simulink model "PDQuadrotor_with_the_position_control"  (R2015b)
settings: Solver=VariableStepAuto  StartTime=start_simulation_drone  StopTime=end_simulation_drone  RelTol=1e-3
values from neighbouring files (symbols this model uses):
  b = 3.13*10^(-5)    (= 3.13e-05)    [drone_parameters.m]    (also in simulazione_sistema.m)
  C_10 = 0.5    [controller_parameters.m]    (also in controller_paramters.m; simulazione_sistema.m)
  C_11 = 2    [controller_parameters.m]    (also in controller_paramters.m; simulazione_sistema.m)
  C_12 = 0.5    [controller_parameters.m]    (also in controller_paramters.m; simulazione_sistema.m)
  C_9 = 2    [controller_parameters.m]    (also in controller_paramters.m; simulazione_sistema.m)
  chi_5_pre = 0    [controller_parameters.m]    (also in controller_paramters.m; drone_model.m = chi_5(end))
  chi_6_pre = 0    [controller_parameters.m]    (also in controller_paramters.m; drone_model.m = chi_6(end))
  d = 7.5*10^(-7)    (= 7.5e-07)    [drone_parameters.m]    (also in simulazione_sistema.m)
  g = 9.81    [drone_parameters.m]    (also in simulazione_sistema.m)
  Ix = 7.5*10^(-3)    (= 0.0075)    [drone_parameters.m]    (also in simulazione_sistema.m)
  Iy = 7.5*10^(-3)    (= 0.0075)    [drone_parameters.m]    (also in simulazione_sistema.m)
  Iz = 1.3*10^(-2)    (= 0.013)    [drone_parameters.m]    (also in simulazione_sistema.m)
  Jr = 6.5*10^(-5)    (= 6.5e-05)    [drone_parameters.m]    (also in simulazione_sistema.m)
  kdp = 0.4e1    (= 4)    [controller_parameters.m]    (also in controller_paramters.m; simulazione_sistema.m)
  kdps = 0.4e1    (= 4)    [controller_parameters.m]    (also in controller_paramters.m; simulazione_sistema.m)
  kdt = 0.4e1    (= 4)    [controller_parameters.m]    (also in controller_paramters.m; simulazione_sistema.m)
  kdz = 20e1    (= 200)    [controller_parameters.m]    (also in controller_paramters.m; simulazione_sistema.m)
  kpp = 0.8e1    (= 8)    [controller_parameters.m]    (also in controller_paramters.m; simulazione_sistema.m)
  kpps = 1e1    (= 10)    [controller_parameters.m]    (also in controller_paramters.m; simulazione_sistema.m)
  kpt = 1.2e1    (= 12)    [controller_parameters.m]    (also in controller_paramters.m; simulazione_sistema.m)
  kpz = 100e1    (= 1000)    [controller_parameters.m]    (also in controller_paramters.m; simulazione_sistema.m)
  l = 0.23    [drone_parameters.m]    (also in simulazione_sistema.m)
  lambda_5 = 0.025    [controller_parameters.m]    (also in controller_paramters.m; simulazione_sistema.m)
  lambda_6 = 0.025    [controller_parameters.m]    (also in controller_paramters.m; simulazione_sistema.m)
  m = 0.65    [drone_parameters.m]    (also in simulazione_sistema.m)
  phi_dot_pre = 0    [controller_parameters.m]    (also in controller_paramters.m; drone_model.m = phi_dot(end))
  pitch_regulator_pre = pitch_initial    [controller_parameters.m]    (also in controller_paramters.m)
  psi_dot_pre = 0    [controller_parameters.m]    (also in controller_paramters.m; drone_model.m = psi_dot(end))
  roll_regulator_pre = roll_initial    [controller_parameters.m]    (also in controller_paramters.m)
  theta_dot_pre = 0    [controller_parameters.m]    (also in controller_paramters.m; drone_model.m = theta_dot(end))
  x_dot_pre = 0    [controller_parameters.m]    (also in drone_model.m = x_dot(end))
  x_next_drone = x_next    [drone_model.m]
  x_next_pre = x_next    [controller_parameters.m]    (also in drone_model.m = x_meas(end))
  y_dot_pre = 0    [controller_parameters.m]    (also in drone_model.m = y_dot(end))
  y_next_drone = -z_next    [drone_model.m]
  y_next_pre = -z_next    [controller_parameters.m]    (also in drone_model.m = y_meas(end))
  yaw_regulator = delta_yaw_regulator + yaw_initial    [drone_control.m]
  yaw_regulator_pre = yaw_initial    [controller_parameters.m]    (also in controller_paramters.m)
  z_dot_pre = 0    [controller_parameters.m]    (also in drone_model.m = z_dot(end))
  z_next_drone = y_next    [drone_model.m]
  z_next_pre = y_next    [controller_parameters.m]    (also in drone_model.m = z_meas(end))
settings Model: Creator=Giuseppe  LastModifiedBy=giuse

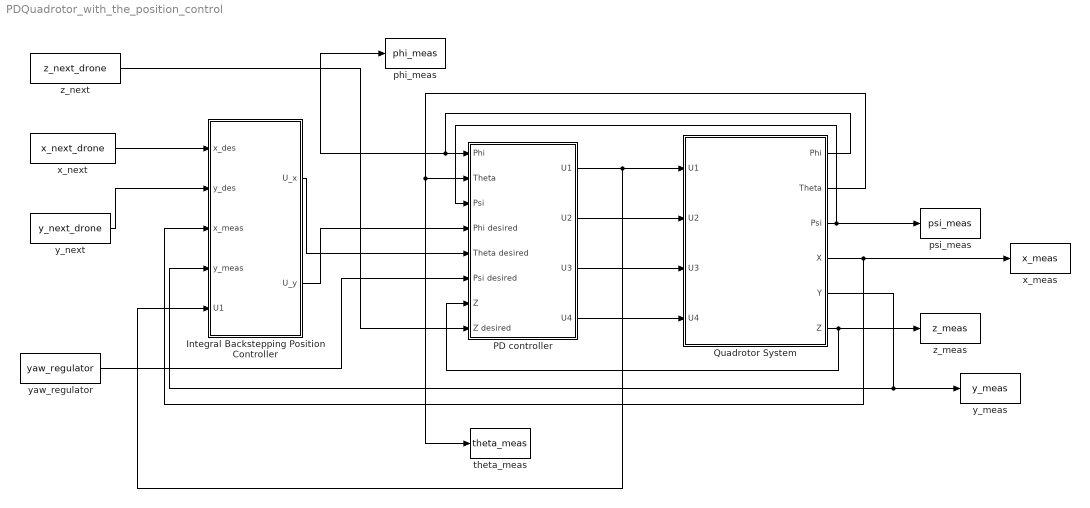
== system PDQuadrotor_with_the_position_control ==
  Integral Backstepping Position Controller : Subsystem
  PD controller : Subsystem
  Quadrotor System : Subsystem
  phi_meas : ToWorkspace  VariableName=phi_meas  SampleTime=-1
  psi_meas : ToWorkspace  VariableName=psi_meas  SampleTime=-1
  theta_meas : ToWorkspace  VariableName=theta_meas  SampleTime=-1
  "x_meas " : ToWorkspace  VariableName=x_meas  SampleTime=-1
  x_next : Constant  Value=x_next_drone
  y_meas : ToWorkspace  VariableName=y_meas  SampleTime=-1
  y_next : Constant  Value=y_next_drone
  yaw_regulator : Constant  Value=yaw_regulator
  z_meas : ToWorkspace  VariableName=z_meas  SampleTime=-1
  z_next : Constant  Value=z_next_drone
  wires:
  PD controller/1(U1) -> Integral Backstepping Position Controller/5(U1), Quadrotor System/1(U1)
  PD controller/2(U2) -> Quadrotor System/2(U2)
  PD controller/3(U3) -> Quadrotor System/3(U3)
  PD controller/4(U4) -> Quadrotor System/4(U4)
  Quadrotor System/6(Z) -> PD controller/7(Z), z_meas/1
  Quadrotor System/1(Phi) -> PD controller/1(Phi), phi_meas/1
  Quadrotor System/2(Theta) -> theta_meas/1, PD controller/2(Theta)
  Quadrotor System/3(Psi) -> PD controller/3(Psi), psi_meas/1
  Integral Backstepping Position Controller/2(U_y) -> PD controller/4(Phi desired)
  Integral Backstepping Position Controller/1(U_x) -> PD controller/5(Theta desired)
  z_next/1 -> PD controller/8(Z desired)
  Quadrotor System/5(Y) -> Integral Backstepping Position Controller/4(y_meas), y_meas/1
  yaw_regulator/1 -> PD controller/6(Psi desired)
  y_next/1 -> Integral Backstepping Position Controller/2(y_des)
  x_next/1 -> Integral Backstepping Position Controller/1(x_des)
  Quadrotor System/4(X) -> Integral Backstepping Position Controller/3(x_meas), "x_meas "/1

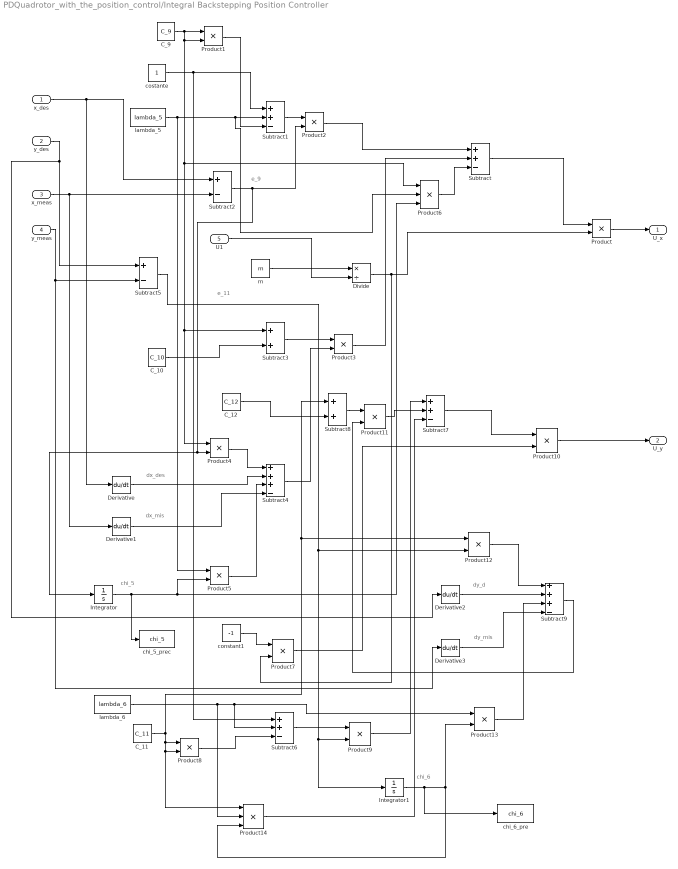
== system PDQuadrotor_with_the_position_control/Integral Backstepping Position Controller ==
  note: chi_6
  note: dy_mis
  note: dy_d
  note: e_11
  note: chi_5
  note: dx_des
  note: dx_mis
  note: e_9
  x_des : Inport
  y_des : Inport  Port=2
  x_meas : Inport  Port=3
  y_meas : Inport  Port=4
  U1 : Inport  Port=5
  C_10 : Constant  Value=C_10
  C_11 : Constant  Value=C_11
  C_12 : Constant  Value=C_12
  C_9 : Constant  Value=C_9
  Derivative{,1..3} (4 alike) : Derivative
  Divide : Product  Inputs=*/
  Integrator : Integrator  InitialCondition=chi_5_pre
  Integrator1 : Integrator  InitialCondition=chi_6_pre
  Product{,1..5,7..13} (13 alike) : Product
  Product14 : Product  Inputs=3
  Product6 : Product  Inputs=3
  Subtract{,1,6..7} (4 alike) : Sum  Inputs=++-
  Subtract2 : Sum  Inputs=+-
  Subtract3 : Sum
  Subtract4 : Sum  Inputs=+++-
  Subtract5 : Sum  Inputs=+-
  Subtract8 : Sum
  Subtract9 : Sum  Inputs=+++-
  chi_5_prec : ToWorkspace  VariableName=chi_5  SampleTime=-1
  chi_6_pre : ToWorkspace  VariableName=chi_6  SampleTime=-1
  constant1 : Constant  Value=-1
  costante : Constant
  lambda_5 : Constant  Value=lambda_5
  lambda_6 : Constant  Value=lambda_6
  m : Constant  Value=m
  U_x : Outport
  U_y : Outport  Port=2
  wires:
  m/1 -> Divide/1
  U1/1 -> Divide/2
  Divide/1 -> Product7/2, Product/2
  Subtract/1 -> Product/1
  costante/1 -> Subtract6/1, Subtract1/1
  lambda_5/1 -> Product6/2, Subtract1/2, Product5/1
  C_9/1 -> Product6/1, Subtract3/1, Product4/1, Product1/2, Product1/1
  Product1/1 -> Subtract1/3
  Subtract1/1 -> Product2/1
  Subtract2/1 -> Integrator/1, Product4/2, Product2/2
  x_des/1 -> Derivative/1, Subtract2/1
  x_meas/1 -> Derivative1/1, Subtract2/2
  Product2/1 -> Subtract/1
  Subtract3/1 -> Product3/1
  C_10/1 -> Subtract3/2
  Subtract4/1 -> Product3/2
  Product4/1 -> Subtract4/1
  Derivative/1 -> Subtract4/2
  Derivative1/1 -> Subtract4/4
  Product5/1 -> Subtract4/3
  Integrator/1 -> chi_5_prec/1, Product6/3, Product5/2
  Product3/1 -> Subtract/2
  Product/1 -> U_x/1
  Product6/1 -> Subtract/3
  constant1/1 -> Product7/1
  C_11/1 -> Product12/1, Subtract8/1, Product14/1, Product8/2, Product8/1
  Product8/1 -> Subtract6/3
  lambda_6/1 -> Product14/2, Subtract6/2, Product13/1
  Subtract6/1 -> Product9/1
  y_des/1 -> Subtract5/1, Derivative2/1
  y_meas/1 -> Subtract5/2, Derivative3/1
  Subtract5/1 -> Product12/2, Product9/2, Integrator1/1
  Product10/1 -> U_y/1
  Subtract7/1 -> Product10/1
  Product7/1 -> Product10/2
  Product9/1 -> Subtract7/1
  C_12/1 -> Subtract8/2
  Subtract8/1 -> Product11/1
  Product11/1 -> Subtract7/2
  Subtract9/1 -> Product11/2
  Product12/1 -> Subtract9/1
  Derivative2/1 -> Subtract9/2
  Derivative3/1 -> Subtract9/4
  Product13/1 -> Subtract9/3
  Integrator1/1 -> chi_6_pre/1, Product14/3, Product13/2
  Product14/1 -> Subtract7/3

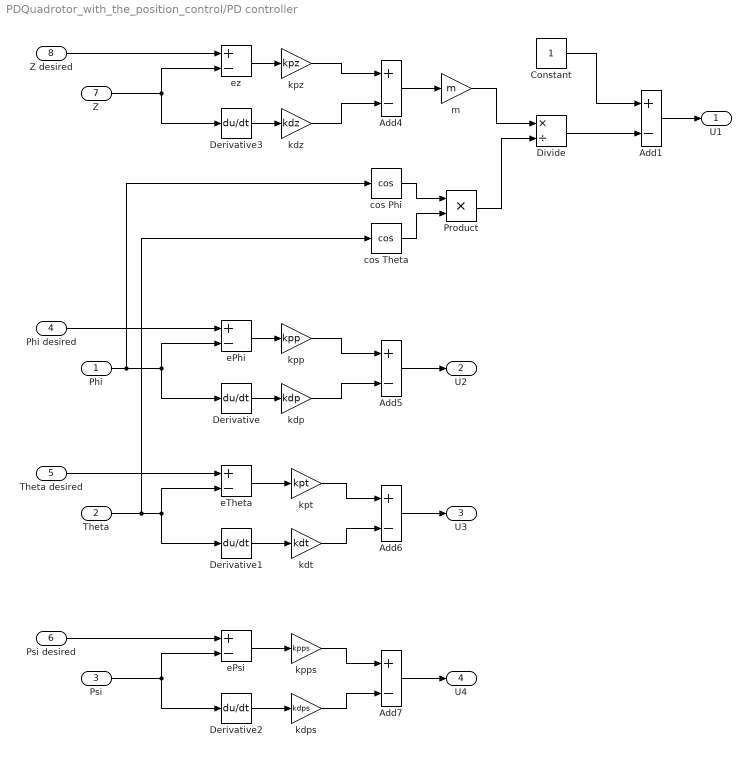
== system PDQuadrotor_with_the_position_control/PD controller ==
  Phi : Inport
  Theta : Inport  Port=2
  Psi : Inport  Port=3
  Phi desired : Inport  Port=4
  Theta desired : Inport  Port=5
  Psi desired : Inport  Port=6
  Z : Inport  Port=7
  Z desired : Inport  Port=8
  Add{1,4..7} (5 alike) : Sum  Inputs=+-
  Constant : Constant
  Derivative{,1..3} (4 alike) : Derivative
  Divide : Product  Inputs=*/
  Product : Product  RndMeth=Zero
  cos Phi : Trigonometry  Operator=cos
  cos Theta : Trigonometry  Operator=cos
  ePhi : Sum  Inputs=+-
  ePsi : Sum  Inputs=+-
  eTheta : Sum  Inputs=+-
  ez : Sum  Inputs=+-
  kdp : Gain  Gain=kdp
  kdps : Gain  Gain=kdps
  kdt : Gain  Gain=kdt
  kdz : Gain  Gain=kdz
  kpp : Gain  Gain=kpp
  kpps : Gain  Gain=kpps
  kpt : Gain  Gain=kpt
  kpz : Gain  Gain=kpz
  m : Gain  Gain=m
  U1 : Outport
  U2 : Outport  Port=2
  U3 : Outport  Port=3
  U4 : Outport  Port=4
  wires:
  Phi/1 -> Derivative/1, ePhi/2, cos Phi/1
  Theta/1 -> Derivative1/1, eTheta/2, cos Theta/1
  Psi/1 -> Derivative2/1, ePsi/2
  Phi desired/1 -> ePhi/1
  Theta desired/1 -> eTheta/1
  Psi desired/1 -> ePsi/1
  ePhi/1 -> kpp/1
  Derivative/1 -> kdp/1
  eTheta/1 -> kpt/1
  Derivative1/1 -> kdt/1
  ePsi/1 -> kpps/1
  Derivative2/1 -> kdps/1
  Z/1 -> Derivative3/1, ez/2
  Z desired/1 -> ez/1
  ez/1 -> kpz/1
  Derivative3/1 -> kdz/1
  kpz/1 -> Add4/1
  kdz/1 -> Add4/2
  kpp/1 -> Add5/1
  kdp/1 -> Add5/2
  Add5/1 -> U2/1
  kpt/1 -> Add6/1
  kdt/1 -> Add6/2
  Add6/1 -> U3/1
  kpps/1 -> Add7/1
  kdps/1 -> Add7/2
  Add7/1 -> U4/1
  cos Phi/1 -> Product/1
  cos Theta/1 -> Product/2
  Add4/1 -> m/1
  m/1 -> Divide/1
  Product/1 -> Divide/2
  Constant/1 -> Add1/1
  Divide/1 -> Add1/2
  Add1/1 -> U1/1

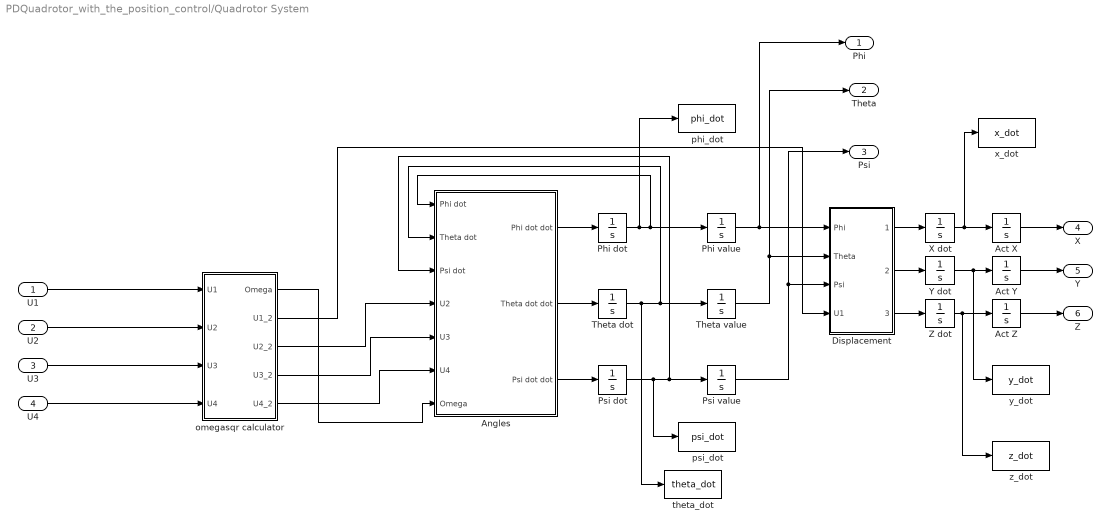
== system PDQuadrotor_with_the_position_control/Quadrotor System ==
  U1 : Inport
  U2 : Inport  Port=2
  U3 : Inport  Port=3
  U4 : Inport  Port=4
  Act X : Integrator  InitialCondition=x_next_pre
  Act Y : Integrator  InitialCondition=y_next_pre
  Act Z : Integrator  InitialCondition=z_next_pre
  Angles : Subsystem
  Displacement : Subsystem
  Phi dot : Integrator  InitialCondition=phi_dot_pre
  Phi value : Integrator  InitialCondition=roll_regulator_pre  ZeroCross=off
  Psi dot : Integrator  InitialCondition=psi_dot_pre  ZeroCross=off
  Psi value : Integrator  InitialCondition=yaw_regulator_pre  ZeroCross=off
  Theta dot : Integrator  InitialCondition=theta_dot_pre  ZeroCross=off
  Theta value : Integrator  InitialCondition=pitch_regulator_pre  ZeroCross=off
  X dot : Integrator  InitialCondition=x_dot_pre
  Y dot : Integrator  InitialCondition=y_dot_pre
  Z dot : Integrator  InitialCondition=z_dot_pre
  omegasqr calculator : Subsystem
  phi_dot : ToWorkspace  VariableName=phi_dot  SampleTime=-1
  psi_dot : ToWorkspace  VariableName=psi_dot  SampleTime=-1
  theta_dot : ToWorkspace  VariableName=theta_dot  SampleTime=-1
  x_dot : ToWorkspace  VariableName=x_dot  SampleTime=-1
  y_dot : ToWorkspace  VariableName=y_dot  SampleTime=-1
  z_dot : ToWorkspace  VariableName=z_dot  SampleTime=-1
  Phi : Outport
  Theta : Outport  Port=2
  Psi : Outport  Port=3
  X : Outport  Port=4
  Y : Outport  Port=5
  Z : Outport  Port=6
  wires:
  Angles/1(Phi dot dot) -> Phi dot/1
  Angles/2(Theta dot dot) -> Theta dot/1
  Angles/3(Psi dot dot) -> Psi dot/1
  Phi dot/1 -> Phi value/1, Angles/1(Phi dot), phi_dot/1
  Theta dot/1 -> Theta value/1, Angles/2(Theta dot), theta_dot/1
  Psi dot/1 -> Psi value/1, Angles/3(Psi dot), psi_dot/1
  omegasqr calculator/3(U2_2) -> Angles/4(U2)
  omegasqr calculator/4(U3_2) -> Angles/5(U3)
  omegasqr calculator/5(U4_2) -> Angles/6(U4)
  omegasqr calculator/1(Omega) -> Angles/7(Omega)
  Phi value/1 -> Displacement/1(Phi), Phi/1
  Theta value/1 -> Displacement/2(Theta), Theta/1
  Psi value/1 -> Displacement/3(Psi), Psi/1
  omegasqr calculator/2(U1_2) -> Displacement/4(U1)
  Displacement/1(x dotdot) -> X dot/1
  X dot/1 -> x_dot/1, Act X/1
  Y dot/1 -> y_dot/1, Act Y/1
  Displacement/2(y dotdot) -> Y dot/1
  Z dot/1 -> z_dot/1, Act Z/1
  Displacement/3(z dotdot) -> Z dot/1
  Act X/1 -> X/1
  Act Y/1 -> Y/1
  Act Z/1 -> Z/1
  U1/1 -> omegasqr calculator/1(U1)
  U2/1 -> omegasqr calculator/2(U2)
  U3/1 -> omegasqr calculator/3(U3)
  U4/1 -> omegasqr calculator/4(U4)

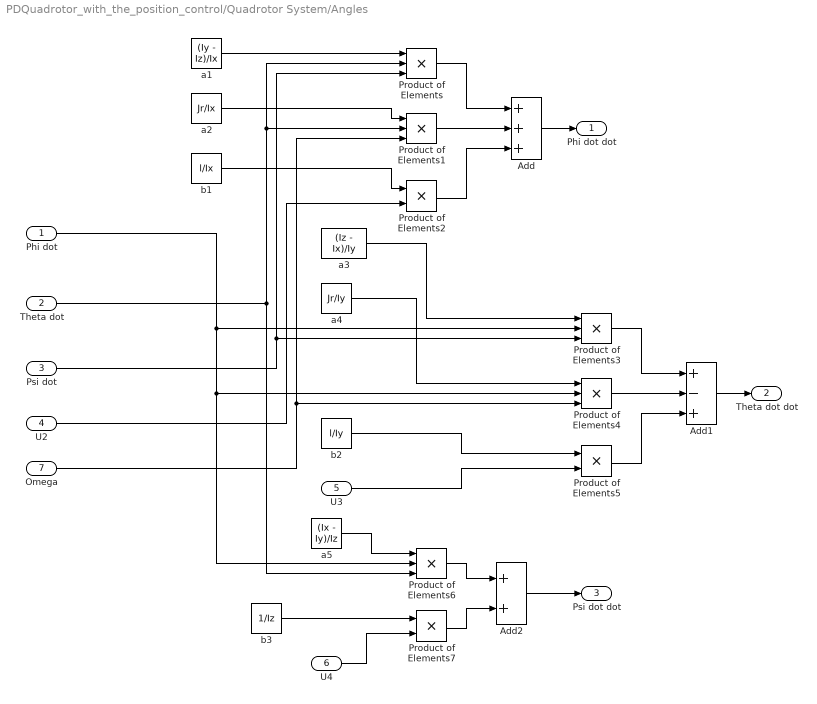
== system PDQuadrotor_with_the_position_control/Quadrotor System/Angles ==
  Phi dot : Inport
  Theta dot : Inport  Port=2
  Psi dot : Inport  Port=3
  U2 : Inport  Port=4
  U3 : Inport  Port=5
  U4 : Inport  Port=6
  Omega : Inport  Port=7
  Add : Sum  Inputs=+++
  Add1 : Sum  Inputs=+-+
  Add2 : Sum
  Product of Elements{,1,3..4,6} (5 alike) : Product  Inputs=3
  Product of Elements2 : Product
  Product of Elements5 : Product
  Product of Elements7 : Product
  a1 : Constant  Value=(Iy - Iz)/Ix
  a2 : Constant  Value=Jr/Ix
  a3 : Constant  Value=(Iz - Ix)/Iy
  a4 : Constant  Value=Jr/Iy
  a5 : Constant  Value=(Ix - Iy)/Iz
  b1 : Constant  Value=l/Ix
  b2 : Constant  Value=l/Iy
  b3 : Constant  Value=1/Iz
  Phi dot dot : Outport
  Theta dot dot : Outport  Port=2
  Psi dot dot : Outport  Port=3
  wires:
  Product of Elements/1 -> Add/1
  Product of Elements1/1 -> Add/2
  Product of Elements2/1 -> Add/3
  Add/1 -> Phi dot dot/1
  a1/1 -> Product of Elements/1
  Theta dot/1 -> Product of Elements/2, Product of Elements1/2, Product of Elements6/3
  Psi dot/1 -> Product of Elements/3, Product of Elements3/3
  a2/1 -> Product of Elements1/1
  b1/1 -> Product of Elements2/1
  U2/1 -> Product of Elements2/2
  Omega/1 -> Product of Elements1/3, Product of Elements4/3
  Product of Elements3/1 -> Add1/1
  Product of Elements4/1 -> Add1/2
  Product of Elements5/1 -> Add1/3
  Add1/1 -> Theta dot dot/1
  a3/1 -> Product of Elements3/1
  a4/1 -> Product of Elements4/1
  b2/1 -> Product of Elements5/1
  U3/1 -> Product of Elements5/2
  Phi dot/1 -> Product of Elements3/2, Product of Elements4/2, Product of Elements6/2
  Product of Elements6/1 -> Add2/1
  Product of Elements7/1 -> Add2/2
  Add2/1 -> Psi dot dot/1
  U4/1 -> Product of Elements7/2
  b3/1 -> Product of Elements7/1
  a5/1 -> Product of Elements6/1

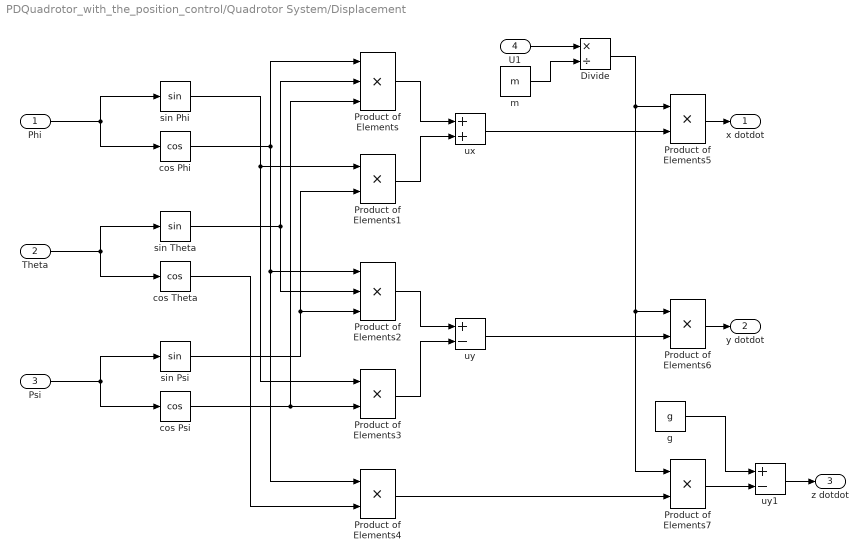
== system PDQuadrotor_with_the_position_control/Quadrotor System/Displacement ==
  Phi : Inport
  Theta : Inport  Port=2
  Psi : Inport  Port=3
  U1 : Inport  Port=4
  Divide : Product  Inputs=*/
  Product of Elements : Product  Inputs=3
  Product of Elements{1,3..7} (6 alike) : Product
  Product of Elements2 : Product  Inputs=3
  cos Phi : Trigonometry  Operator=cos
  cos Psi : Trigonometry  Operator=cos
  cos Theta : Trigonometry  Operator=cos
  g : Constant  Value=g
  m : Constant  Value=m
  sin Phi : Trigonometry
  sin Psi : Trigonometry
  sin Theta : Trigonometry
  ux : Sum
  uy : Sum  Inputs=+-
  uy1 : Sum  Inputs=+-
  x dotdot : Outport
  y dotdot : Outport  Port=2
  z dotdot : Outport  Port=3
  wires:
  Phi/1 -> sin Phi/1, cos Phi/1
  Theta/1 -> sin Theta/1, cos Theta/1
  Psi/1 -> sin Psi/1, cos Psi/1
  sin Theta/1 -> Product of Elements/2, Product of Elements2/2
  cos Psi/1 -> Product of Elements/3, Product of Elements3/2
  cos Phi/1 -> Product of Elements/1, Product of Elements2/1, Product of Elements4/1
  sin Phi/1 -> Product of Elements1/1, Product of Elements3/1
  sin Psi/1 -> Product of Elements1/2, Product of Elements2/3
  Product of Elements/1 -> ux/1
  Product of Elements1/1 -> ux/2
  ux/1 -> Product of Elements5/2
  Product of Elements2/1 -> uy/1
  Product of Elements3/1 -> uy/2
  uy/1 -> Product of Elements6/2
  cos Theta/1 -> Product of Elements4/2
  Product of Elements4/1 -> Product of Elements7/2
  U1/1 -> Divide/1
  m/1 -> Divide/2
  Divide/1 -> Product of Elements5/1, Product of Elements6/1, Product of Elements7/1
  Product of Elements5/1 -> x dotdot/1
  Product of Elements6/1 -> y dotdot/1
  uy1/1 -> z dotdot/1
  Product of Elements7/1 -> uy1/2
  g/1 -> uy1/1

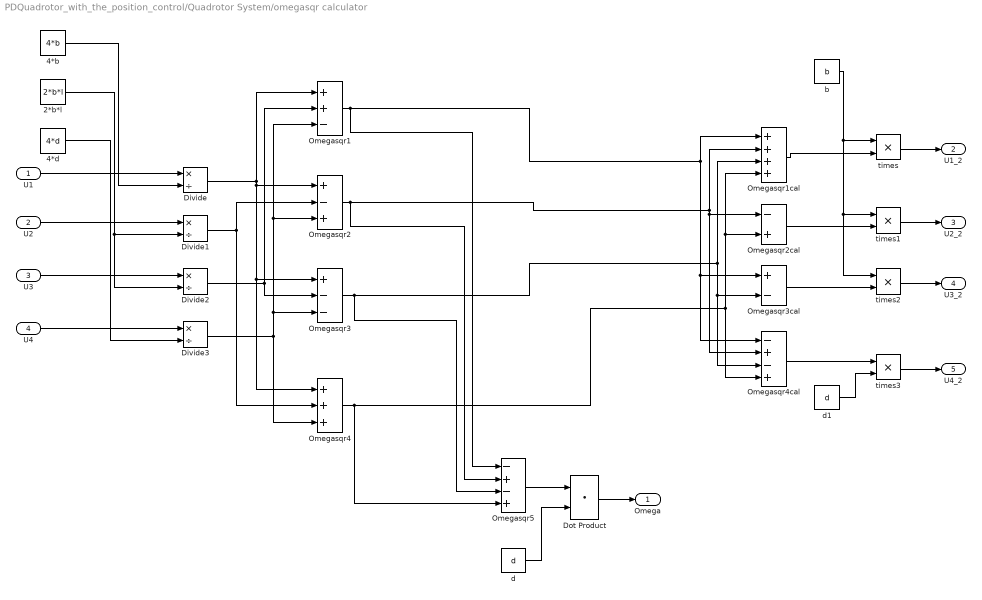
== system PDQuadrotor_with_the_position_control/Quadrotor System/omegasqr calculator ==
  U1 : Inport
  U2 : Inport  Port=2
  U3 : Inport  Port=3
  U4 : Inport  Port=4
  2*b*l : Constant  Value=2*b*l
  4*b : Constant  Value=4*b
  4*d : Constant  Value=4*d
  Divide{,1..3} (4 alike) : Product  Inputs=*/
  Dot Product : DotProduct  InputSameDT=on  OutDataTypeStr=Inherit: Inherit via internal rule
  Omegasqr1 : Sum  Inputs=++-
  Omegasqr1cal : Sum  Inputs=++++
  Omegasqr2 : Sum  Inputs=+-+
  Omegasqr2cal : Sum  Inputs=-+
  Omegasqr3 : Sum  Inputs=+--
  Omegasqr3cal : Sum  Inputs=+-
  Omegasqr4 : Sum  Inputs=+++
  Omegasqr4cal : Sum  Inputs=-+-+
  Omegasqr5 : Sum  Inputs=-+-+
  b : Constant  Value=b
  d : Constant  Value=d
  d1 : Constant  Value=d
  times{,1..3} (4 alike) : Product  Inputs=**
  Omega : Outport
  U1_2 : Outport  Port=2
  U2_2 : Outport  Port=3
  U3_2 : Outport  Port=4
  U4_2 : Outport  Port=5
  wires:
  U1/1 -> Divide/1
  4*b/1 -> Divide/2
  U2/1 -> Divide1/1
  2*b*l/1 -> Divide1/2, Divide2/2
  U3/1 -> Divide2/1
  U4/1 -> Divide3/1
  4*d/1 -> Divide3/2
  Divide/1 -> Omegasqr1/1, Omegasqr2/1, Omegasqr3/1, Omegasqr4/1
  Divide2/1 -> Omegasqr1/2, Omegasqr3/2
  Divide3/1 -> Omegasqr1/3, Omegasqr2/3, Omegasqr3/3, Omegasqr4/3
  Divide1/1 -> Omegasqr2/2, Omegasqr4/2
  Omegasqr1/1 -> Omegasqr5/1, Omegasqr1cal/1, Omegasqr3cal/1, Omegasqr4cal/1
  Omegasqr2/1 -> Omegasqr5/2, Omegasqr1cal/2, Omegasqr2cal/1, Omegasqr4cal/2
  Omegasqr3/1 -> Omegasqr5/3, Omegasqr1cal/3, Omegasqr3cal/2, Omegasqr4cal/3
  Omegasqr4/1 -> Omegasqr5/4, Omegasqr1cal/4, Omegasqr2cal/2, Omegasqr4cal/4
  Omegasqr5/1 -> Dot Product/1
  Dot Product/1 -> Omega/1
  d/1 -> Dot Product/2
  b/1 -> times/1, times1/1, times2/1
  Omegasqr1cal/1 -> times/2
  Omegasqr2cal/1 -> times1/2
  Omegasqr3cal/1 -> times2/2
  Omegasqr4cal/1 -> times3/1
  d1/1 -> times3/2
  times/1 -> U1_2/1
  times1/1 -> U2_2/1
  times3/1 -> U4_2/1
  times2/1 -> U3_2/1
